simulink library "inp"  (R2021b)
settings: Solver=VariableStepAuto  StartTime=0.0  StopTime=10.0  RelTol=1e-3
undefined symbols (not defined in the file): C_TASK_5MS_S, FALSE, KINP_AcoreReadyToSlp_flg_ovrdflg, KINP_AcoreReadyToSlp_flg_ovrdval, KINP_AllowMovThd_OTA_enum_ovrdflg, KINP_AllowMovThd_OTA_enum_ovrdval, KINP_APSAngleTarget_Deg_ovrdflg, KINP_APSAngleTarget_Deg_ovrdval, KINP_APSDecReq_mps2_ovrdflg, KINP_APSDecReq_mps2_ovrdval, KINP_APSDecReqA_flg_ovrdflg, KINP_APSDecReqA_flg_ovrdval, KINP_APSDFLL_cm_ovrdflg, KINP_APSDFLL_cm_ovrdval, KINP_APSDFLR_cm_ovrdflg, KINP_APSDFLR_cm_ovrdval, KINP_APSDRLL_cm_ovrdflg, KINP_APSDRLL_cm_ovrdval, KINP_APSDRLR_cm_ovrdflg, KINP_APSDRLR_cm_ovrdval, KINP_APSExitCondition_enum_ovrdflg, KINP_APSExitCondition_enum_ovrdval, KINP_APSHWVer_enum_ovrdflg, KINP_APSHWVer_enum_ovrdval, KINP_APSProgressPCT_pct_ovrdflg, KINP_APSProgressPCT_pct_ovrdval, KINP_APSReq_enum_ovrdflg, KINP_APSReq_enum_ovrdval, KINP_APSRQDisplay_enum_ovrdflg, KINP_APSRQDisplay_enum_ovrdval, KINP_APSRqEPASCtrl_flg_ovrdflg, KINP_APSRqEPASCtrl_flg_ovrdval, KINP_APSShiftPosnReq_enum_ovrdval, KINP_APSShiftPosnReq_enum_ovrflg, KINP_APSSpeedCMD_kph_ovrdval, KINP_APSSpeedCMD_kph_ovrflg, KINP_APSStaSystem_enum_ovrdflg, KINP_APSStaSystem_enum_ovrdval, KINP_APSSWVer_enum_ovrdflg, KINP_APSSWVer_enum_ovrdval, KINP_APSVMCReqA_flg_ovrdval, KINP_APSVMCReqA_flg_ovrflg, KINP_APSVRqEPASCtrl_flg_ovrdflg, KINP_APSVRqEPASCtrl_flg_ovrdval, KINP_AuxBattVolmV_mV_ovrdflg, KINP_AuxBattVolmV_mV_ovrdval, KINP_CAASSta_enum_ovrdflg, KINP_CAASSta_enum_ovrdval, KINP_CAASVMCReqA_flg_ovrdval, KINP_CAASVMCReqA_flg_ovrflg, KINP_Chime_enum_ovrdflg, KINP_Chime_enum_ovrdval, KINP_ClearDTCcmd_flg_ovrdflg, KINP_ClearDTCcmd_flg_ovrdval, KINP_EvccAplusPwrUpReq_flg_ovrdflg, KINP_EvccAplusPwrUpReq_flg_ovrdval, KINP_LFID_raw_ovrdval, KINP_LFID_raw_ovrflg, KINP_LRID_raw_ovrdval, KINP_MemOffsetAccX_raw16_ovrdflg ... (+118)
libraries: FVT_lib x595, hcu_lib x1
(part 23 of 27)

== system inp/INP/CAN4/SignalCheck/GW_ZoneDR1 ==
  BHAL_outputs : Inport
  inp_CanValid_bus : Inport  Port=2
  CSWDimSw : FVT_lib/inp/can_signal_template  SystemSampleTime=-1  VariantActivationTime=update diagram  Latency=0  AutoFrameSizeCalculation=off
      link override defval: Value=KINP_CSWDimSw_flg_defval
      link override fftdec: Value=KINP_CSWDimSw_flg_fftdec
      link override fftinc: Value=KINP_CSWDimSw_flg_fftinc
      link override fftlim: Value=KINP_CSWDimSw_flg_fftlim
      link override invalid: Value=KINP_CSWDimSw_flg_invalid
      link override ovrdflg: Value=KINP_CSWDimSw_flg_ovrdflg
      link override ovrdval: Value=KINP_CSWDimSw_flg_ovrdval
      link override setvalid: Value=KINP_CSWDimSw_flg_setvalid
      link override srvcflg: Value=KINP_CSWDimSw_flg_srvcflg
      link override srvcval: Value=KINP_CSWDimSw_flg_srvcval
  CSWFWasSwSta : FVT_lib/inp/can_signal_template  SystemSampleTime=-1  VariantActivationTime=update diagram  Latency=0  AutoFrameSizeCalculation=off
      link override defval: Value=KINP_CSWFWasSwSta_enum_defval
      link override fftdec: Value=KINP_CSWFWasSwSta_enum_fftdec
      link override fftinc: Value=KINP_CSWFWasSwSta_enum_fftinc
      link override fftlim: Value=KINP_CSWFWasSwSta_enum_fftlim
      link override invalid: Value=KINP_CSWFWasSwSta_enum_invalid
      link override ovrdflg: Value=KINP_CSWFWasSwSta_enum_ovrdflg
      link override ovrdval: Value=KINP_CSWFWasSwSta_enum_ovrdval
      link override setvalid: Value=KINP_CSWFWasSwSta_enum_setvalid
      link override srvcflg: Value=KINP_CSWFWasSwSta_enum_srvcflg
      link override srvcval: Value=KINP_CSWFWasSwSta_enum_srvcval
  CSWFWipSwSta : FVT_lib/inp/can_signal_template  SystemSampleTime=-1  VariantActivationTime=update diagram  Latency=0  AutoFrameSizeCalculation=off
      link override defval: Value=KINP_CSWFWipSwSta_enum_defval
      link override fftdec: Value=KINP_CSWFWipSwSta_enum_fftdec
      link override fftinc: Value=KINP_CSWFWipSwSta_enum_fftinc
      link override fftlim: Value=KINP_CSWFWipSwSta_enum_fftlim
      link override invalid: Value=KINP_CSWFWipSwSta_enum_invalid
      link override ovrdflg: Value=KINP_CSWFWipSwSta_enum_ovrdflg
      link override ovrdval: Value=KINP_CSWFWipSwSta_enum_ovrdval
      link override setvalid: Value=KINP_CSWFWipSwSta_enum_setvalid
      link override srvcflg: Value=KINP_CSWFWipSwSta_enum_srvcflg
      link override srvcval: Value=KINP_CSWFWipSwSta_enum_srvcval
  CSWPassSWSta : FVT_lib/inp/can_signal_template  SystemSampleTime=-1  VariantActivationTime=update diagram  Latency=0  AutoFrameSizeCalculation=off
      link override defval: Value=KINP_CSWPassSWSta_flg_defval
      link override fftdec: Value=KINP_CSWPassSWSta_flg_fftdec
      link override fftinc: Value=KINP_CSWPassSWSta_flg_fftinc
      link override fftlim: Value=KINP_CSWPassSWSta_flg_fftlim
      link override invalid: Value=KINP_CSWPassSWSta_flg_invalid
      link override ovrdflg: Value=KINP_CSWPassSWSta_flg_ovrdflg
      link override ovrdval: Value=KINP_CSWPassSWSta_flg_ovrdval
      link override setvalid: Value=KINP_CSWPassSWSta_flg_setvalid
      link override srvcflg: Value=KINP_CSWPassSWSta_flg_srvcflg
      link override srvcval: Value=KINP_CSWPassSWSta_flg_srvcval
  CSWRWasSWSta : FVT_lib/inp/can_signal_template  SystemSampleTime=-1  VariantActivationTime=update diagram  Latency=0  AutoFrameSizeCalculation=off
      link override defval: Value=KINP_CSWRWasSWSta_enum_defval
      link override fftdec: Value=KINP_CSWRWasSWSta_enum_fftdec
      link override fftinc: Value=KINP_CSWRWasSWSta_enum_fftinc
      link override fftlim: Value=KINP_CSWRWasSWSta_enum_fftlim
      link override invalid: Value=KINP_CSWRWasSWSta_enum_invalid
      link override ovrdflg: Value=KINP_CSWRWasSWSta_enum_ovrdflg
      link override ovrdval: Value=KINP_CSWRWasSWSta_enum_ovrdval
      link override setvalid: Value=KINP_CSWRWasSWSta_enum_setvalid
      link override srvcflg: Value=KINP_CSWRWasSWSta_enum_srvcflg
      link override srvcval: Value=KINP_CSWRWasSWSta_enum_srvcval
  CSWRWipIntSwSta : FVT_lib/inp/can_signal_template  SystemSampleTime=-1  VariantActivationTime=update diagram  Latency=0  AutoFrameSizeCalculation=off
      link override defval: Value=KINP_CSWRWipIntSwSta_enum_defval
      link override fftdec: Value=KINP_CSWRWipIntSwSta_enum_fftdec
      link override fftinc: Value=KINP_CSWRWipIntSwSta_enum_fftinc
      link override fftlim: Value=KINP_CSWRWipIntSwSta_enum_fftlim
      link override invalid: Value=KINP_CSWRWipIntSwSta_enum_invalid
      link override ovrdflg: Value=KINP_CSWRWipIntSwSta_enum_ovrdflg
      link override ovrdval: Value=KINP_CSWRWipIntSwSta_enum_ovrdval
      link override setvalid: Value=KINP_CSWRWipIntSwSta_enum_setvalid
      link override srvcflg: Value=KINP_CSWRWipIntSwSta_enum_srvcflg
      link override srvcval: Value=KINP_CSWRWipIntSwSta_enum_srvcval
  CSWTurnSwSta : FVT_lib/inp/can_signal_template  SystemSampleTime=-1  VariantActivationTime=update diagram  Latency=0  AutoFrameSizeCalculation=off
      link override defval: Value=KINP_CSWTurnSwSta_enum_defval
      link override fftdec: Value=KINP_CSWTurnSwSta_enum_fftdec
      link override fftinc: Value=KINP_CSWTurnSwSta_enum_fftinc
      link override fftlim: Value=KINP_CSWTurnSwSta_enum_fftlim
      link override invalid: Value=KINP_CSWTurnSwSta_enum_invalid
      link override ovrdflg: Value=KINP_CSWTurnSwSta_enum_ovrdflg
      link override ovrdval: Value=KINP_CSWTurnSwSta_enum_ovrdval
      link override setvalid: Value=KINP_CSWTurnSwSta_enum_setvalid
      link override srvcflg: Value=KINP_CSWTurnSwSta_enum_srvcflg
      link override srvcval: Value=KINP_CSWTurnSwSta_enum_srvcval
  DrLockSta : FVT_lib/inp/can_signal_template  SystemSampleTime=-1  VariantActivationTime=update diagram  Latency=0  AutoFrameSizeCalculation=off
      link override defval: Value=KINP_DrLockSta_flg_defval
      link override fftdec: Value=KINP_DrLockSta_flg_fftdec
      link override fftinc: Value=KINP_DrLockSta_flg_fftinc
      link override fftlim: Value=KINP_DrLockSta_flg_fftlim
      link override invalid: Value=KINP_DrLockSta_flg_invalid
      link override ovrdflg: Value=KINP_DrLockSta_flg_ovrdflg
      link override ovrdval: Value=KINP_DrLockSta_flg_ovrdval
      link override setvalid: Value=KINP_DrLockSta_flg_setvalid
      link override srvcflg: Value=KINP_DrLockSta_flg_srvcflg
      link override srvcval: Value=KINP_DrLockSta_flg_srvcval
  MIRRORFOLDSW : FVT_lib/inp/can_signal_template  SystemSampleTime=-1  VariantActivationTime=update diagram  Latency=0  AutoFrameSizeCalculation=off
      link override defval: Value=KINP_MIRRORFOLDSW_flg_defval
      link override fftdec: Value=KINP_MIRRORFOLDSW_flg_fftdec
      link override fftinc: Value=KINP_MIRRORFOLDSW_flg_fftinc
      link override fftlim: Value=KINP_MIRRORFOLDSW_flg_fftlim
      link override invalid: Value=KINP_MIRRORFOLDSW_flg_invalid
      link override ovrdflg: Value=KINP_MIRRORFOLDSW_flg_ovrdflg
      link override ovrdval: Value=KINP_MIRRORFOLDSW_flg_ovrdval
      link override setvalid: Value=KINP_MIRRORFOLDSW_flg_setvalid
      link override srvcflg: Value=KINP_MIRRORFOLDSW_flg_srvcflg
      link override srvcval: Value=KINP_MIRRORFOLDSW_flg_srvcval
  RLSLampSta : FVT_lib/inp/can_signal_template  SystemSampleTime=-1  VariantActivationTime=update diagram  Latency=0  AutoFrameSizeCalculation=off
      link override defval: Value=KINP_RLSLampSta_flg_defval
      link override fftdec: Value=KINP_RLSLampSta_flg_fftdec
      link override fftinc: Value=KINP_RLSLampSta_flg_fftinc
      link override fftlim: Value=KINP_RLSLampSta_flg_fftlim
      link override invalid: Value=KINP_RLSLampSta_flg_invalid
      link override ovrdflg: Value=KINP_RLSLampSta_flg_ovrdflg
      link override ovrdval: Value=KINP_RLSLampSta_flg_ovrdval
      link override setvalid: Value=KINP_RLSLampSta_flg_setvalid
      link override srvcflg: Value=KINP_RLSLampSta_flg_srvcflg
      link override srvcval: Value=KINP_RLSLampSta_flg_srvcval
  RLSRainSnrWiperCmd : FVT_lib/inp/can_signal_template  SystemSampleTime=-1  VariantActivationTime=update diagram  Latency=0  AutoFrameSizeCalculation=off
      link override defval: Value=KINP_RLSRainSnrWiperCmd_enum_defval
      link override fftdec: Value=KINP_RLSRainSnrWiperCmd_enum_fftdec
      link override fftinc: Value=KINP_RLSRainSnrWiperCmd_enum_fftinc
      link override fftlim: Value=KINP_RLSRainSnrWiperCmd_enum_fftlim
      link override invalid: Value=KINP_RLSRainSnrWiperCmd_enum_invalid
      link override ovrdflg: Value=KINP_RLSRainSnrWiperCmd_enum_ovrdflg
      link override ovrdval: Value=KINP_RLSRainSnrWiperCmd_enum_ovrdval
      link override setvalid: Value=KINP_RLSRainSnrWiperCmd_enum_setvalid
      link override srvcflg: Value=KINP_RLSRainSnrWiperCmd_enum_srvcflg
      link override srvcval: Value=KINP_RLSRainSnrWiperCmd_enum_srvcval
  RLTurnLampC : FVT_lib/inp/can_signal_template  SystemSampleTime=-1  VariantActivationTime=update diagram  Latency=0  AutoFrameSizeCalculation=off
      link override defval: Value=KINP_RLTurnLampC_mA_defval
      link override fftdec: Value=KINP_RLTurnLampC_mA_fftdec
      link override fftinc: Value=KINP_RLTurnLampC_mA_fftinc
      link override fftlim: Value=KINP_RLTurnLampC_mA_fftlim
      link override invalid: Value=KINP_RLTurnLampC_mA_invalid
      link override ovrdflg: Value=KINP_RLTurnLampC_mA_ovrdflg
      link override ovrdval: Value=KINP_RLTurnLampC_mA_ovrdval
      link override setvalid: Value=KINP_RLTurnLampC_mA_setvalid
      link override srvcflg: Value=KINP_RLTurnLampC_mA_srvcflg
      link override srvcval: Value=KINP_RLTurnLampC_mA_srvcval
  RRTurnLampC : FVT_lib/inp/can_signal_template  SystemSampleTime=-1  VariantActivationTime=update diagram  Latency=0  AutoFrameSizeCalculation=off
      link override defval: Value=KINP_RRTurnLampC_mA_defval
      link override fftdec: Value=KINP_RRTurnLampC_mA_fftdec
      link override fftinc: Value=KINP_RRTurnLampC_mA_fftinc
      link override fftlim: Value=KINP_RRTurnLampC_mA_fftlim
      link override invalid: Value=KINP_RRTurnLampC_mA_invalid
      link override ovrdflg: Value=KINP_RRTurnLampC_mA_ovrdflg
      link override ovrdval: Value=KINP_RRTurnLampC_mA_ovrdval
      link override setvalid: Value=KINP_RRTurnLampC_mA_setvalid
      link override srvcflg: Value=KINP_RRTurnLampC_mA_srvcflg
      link override srvcval: Value=KINP_RRTurnLampC_mA_srvcval
  RWiperAS : FVT_lib/inp/can_signal_template  SystemSampleTime=-1  VariantActivationTime=update diagram  Latency=0  AutoFrameSizeCalculation=off
      link override defval: Value=KINP_RWiperAS_flg_defval
      link override fftdec: Value=KINP_RWiperAS_flg_fftdec
      link override fftinc: Value=KINP_RWiperAS_flg_fftinc
      link override fftlim: Value=KINP_RWiperAS_flg_fftlim
      link override invalid: Value=KINP_RWiperAS_flg_invalid
      link override ovrdflg: Value=KINP_RWiperAS_flg_ovrdflg
      link override ovrdval: Value=KINP_RWiperAS_flg_ovrdval
      link override setvalid: Value=KINP_RWiperAS_flg_setvalid
      link override srvcflg: Value=KINP_RWiperAS_flg_srvcflg
      link override srvcval: Value=KINP_RWiperAS_flg_srvcval
  RWiperProtection : FVT_lib/inp/can_signal_template  SystemSampleTime=-1  VariantActivationTime=update diagram  Latency=0  AutoFrameSizeCalculation=off
      link override defval: Value=KINP_RWiperProtection_flg_defval
      link override fftdec: Value=KINP_RWiperProtection_flg_fftdec
      link override fftinc: Value=KINP_RWiperProtection_flg_fftinc
      link override fftlim: Value=KINP_RWiperProtection_flg_fftlim
      link override invalid: Value=KINP_RWiperProtection_flg_invalid
      link override ovrdflg: Value=KINP_RWiperProtection_flg_ovrdflg
      link override ovrdval: Value=KINP_RWiperProtection_flg_ovrdval
      link override setvalid: Value=KINP_RWiperProtection_flg_setvalid
      link override srvcflg: Value=KINP_RWiperProtection_flg_srvcflg
      link override srvcval: Value=KINP_RWiperProtection_flg_srvcval
  Terminator_{1..15} (15 alike) : Terminator
  True_VHAL_CSWDimSw_flg : Constant  Value=TRUE  OutDataTypeStr=boolean
  True_VHAL_CSWFWasSwSta_enum : Constant  Value=TRUE  OutDataTypeStr=boolean
  True_VHAL_CSWFWipSwSta_enum : Constant  Value=TRUE  OutDataTypeStr=boolean
  True_VHAL_CSWPassSWSta_flg : Constant  Value=TRUE  OutDataTypeStr=boolean
  True_VHAL_CSWRWasSWSta_enum : Constant  Value=TRUE  OutDataTypeStr=boolean
  True_VHAL_CSWRWipIntSwSta_enum : Constant  Value=TRUE  OutDataTypeStr=boolean
  True_VHAL_CSWTurnSwSta_enum : Constant  Value=TRUE  OutDataTypeStr=boolean
  True_VHAL_DrLockSta_flg : Constant  Value=TRUE  OutDataTypeStr=boolean
  True_VHAL_MIRRORFOLDSW_flg : Constant  Value=TRUE  OutDataTypeStr=boolean
  True_VHAL_RLSLampSta_flg : Constant  Value=TRUE  OutDataTypeStr=boolean
  True_VHAL_RLSRainSnrWiperCmd_enum : Constant  Value=TRUE  OutDataTypeStr=boolean
  True_VHAL_RLTurnLampC_mA : Constant  Value=TRUE  OutDataTypeStr=boolean
  True_VHAL_RRTurnLampC_mA : Constant  Value=TRUE  OutDataTypeStr=boolean
  True_VHAL_RWiperAS_flg : Constant  Value=TRUE  OutDataTypeStr=boolean
  True_VHAL_RWiperProtection_flg : Constant  Value=TRUE  OutDataTypeStr=boolean
  slr1_{1..15} (15 alike) : BusSelector  OutputSignals=VINP_CANMsgValidGWZoneDR1_flg
  slr_VHAL_CSWDimSw_flg : BusSelector  OutputSignals=VHAL_CSWDimSw_flg
  slr_VHAL_CSWFWasSwSta_enum : BusSelector  OutputSignals=VHAL_CSWFWasSwSta_enum
  slr_VHAL_CSWFWipSwSta_enum : BusSelector  OutputSignals=VHAL_CSWFWipSwSta_enum
  slr_VHAL_CSWPassSWSta_flg : BusSelector  OutputSignals=VHAL_CSWPassSWSta_flg
  slr_VHAL_CSWRWasSWSta_enum : BusSelector  OutputSignals=VHAL_CSWRWasSWSta_enum
  slr_VHAL_CSWRWipIntSwSta_enum : BusSelector  OutputSignals=VHAL_CSWRWipIntSwSta_enum
  slr_VHAL_CSWTurnSwSta_enum : BusSelector  OutputSignals=VHAL_CSWTurnSwSta_enum
  slr_VHAL_DrLockSta_flg : BusSelector  OutputSignals=VHAL_DrLockSta_flg
  slr_VHAL_MIRRORFOLDSW_flg : BusSelector  OutputSignals=VHAL_MIRRORFOLDSW_flg
  slr_VHAL_RLSLampSta_flg : BusSelector  OutputSignals=VHAL_RLSLampSta_flg
  slr_VHAL_RLSRainSnrWiperCmd_enum : BusSelector  OutputSignals=VHAL_RLSRainSnrWiperCmd_enum
  slr_VHAL_RLTurnLampC_mA : BusSelector  OutputSignals=VHAL_RLTurnLampC_mA
  slr_VHAL_RRTurnLampC_mA : BusSelector  OutputSignals=VHAL_RRTurnLampC_mA
  slr_VHAL_RWiperAS_flg : BusSelector  OutputSignals=VHAL_RWiperAS_flg
  slr_VHAL_RWiperProtection_flg : BusSelector  OutputSignals=VHAL_RWiperProtection_flg
  VINP_CSWDimSw_flg : Outport
  VINP_CSWFWasSwSta_enum : Outport  Port=2
  VINP_CSWFWipSwSta_enum : Outport  Port=3
  VINP_CSWPassSWSta_flg : Outport  Port=4
  VINP_CSWRWasSWSta_enum : Outport  Port=5
  VINP_CSWRWipIntSwSta_enum : Outport  Port=6
  VINP_CSWTurnSwSta_enum : Outport  Port=7
  VINP_DrLockSta_flg : Outport  Port=8
  VINP_MIRRORFOLDSW_flg : Outport  Port=9
  VINP_RLSLampSta_flg : Outport  Port=10
  VINP_RLSRainSnrWiperCmd_enum : Outport  Port=11
  VINP_RLTurnLampC_mA : Outport  Port=12
  VINP_RRTurnLampC_mA : Outport  Port=13
  VINP_RWiperAS_flg : Outport  Port=14
  VINP_RWiperProtection_flg : Outport  Port=15
  wires:
  BHAL_outputs/1 -> [BHAL_outputs]
  inp_CanValid_bus/1 -> [inp_CanValid_bus]
  [BHAL_outputs] -> slr_VHAL_CSWDimSw_flg/1
  slr_VHAL_CSWDimSw_flg/1 -> CSWDimSw/1  "<VHAL_CSWDimSw_flg>"
  True_VHAL_CSWDimSw_flg/1 -> CSWDimSw/2
  [inp_CanValid_bus] -> slr1_1/1
  slr1_1/1 -> CSWDimSw/3  "<VINP_CANMsgValidGWZoneDR1_flg>"
  CSWDimSw/1 -> VINP_CSWDimSw_flg/1  "VINP_CSWDimSw_flg"
  CSWDimSw/2 -> Terminator_1/1
  [BHAL_outputs] -> slr_VHAL_CSWFWasSwSta_enum/1
  slr_VHAL_CSWFWasSwSta_enum/1 -> CSWFWasSwSta/1  "<VHAL_CSWFWasSwSta_enum>"
  True_VHAL_CSWFWasSwSta_enum/1 -> CSWFWasSwSta/2
  [inp_CanValid_bus] -> slr1_2/1
  slr1_2/1 -> CSWFWasSwSta/3  "<VINP_CANMsgValidGWZoneDR1_flg>"
  CSWFWasSwSta/1 -> VINP_CSWFWasSwSta_enum/1  "VINP_CSWFWasSwSta_enum"
  CSWFWasSwSta/2 -> Terminator_2/1
  [BHAL_outputs] -> slr_VHAL_CSWFWipSwSta_enum/1
  slr_VHAL_CSWFWipSwSta_enum/1 -> CSWFWipSwSta/1  "<VHAL_CSWFWipSwSta_enum>"
  True_VHAL_CSWFWipSwSta_enum/1 -> CSWFWipSwSta/2
  [inp_CanValid_bus] -> slr1_3/1
  slr1_3/1 -> CSWFWipSwSta/3  "<VINP_CANMsgValidGWZoneDR1_flg>"
  CSWFWipSwSta/1 -> VINP_CSWFWipSwSta_enum/1  "VINP_CSWFWipSwSta_enum"
  CSWFWipSwSta/2 -> Terminator_3/1
  [BHAL_outputs] -> slr_VHAL_CSWPassSWSta_flg/1
  slr_VHAL_CSWPassSWSta_flg/1 -> CSWPassSWSta/1  "<VHAL_CSWPassSWSta_flg>"
  True_VHAL_CSWPassSWSta_flg/1 -> CSWPassSWSta/2
  [inp_CanValid_bus] -> slr1_4/1
  slr1_4/1 -> CSWPassSWSta/3  "<VINP_CANMsgValidGWZoneDR1_flg>"
  CSWPassSWSta/1 -> VINP_CSWPassSWSta_flg/1  "VINP_CSWPassSWSta_flg"
  CSWPassSWSta/2 -> Terminator_4/1
  [BHAL_outputs] -> slr_VHAL_CSWRWasSWSta_enum/1
  slr_VHAL_CSWRWasSWSta_enum/1 -> CSWRWasSWSta/1  "<VHAL_CSWRWasSWSta_enum>"
  True_VHAL_CSWRWasSWSta_enum/1 -> CSWRWasSWSta/2
  [inp_CanValid_bus] -> slr1_5/1
  slr1_5/1 -> CSWRWasSWSta/3  "<VINP_CANMsgValidGWZoneDR1_flg>"
  CSWRWasSWSta/1 -> VINP_CSWRWasSWSta_enum/1  "VINP_CSWRWasSWSta_enum"
  CSWRWasSWSta/2 -> Terminator_5/1
  [BHAL_outputs] -> slr_VHAL_CSWRWipIntSwSta_enum/1
  slr_VHAL_CSWRWipIntSwSta_enum/1 -> CSWRWipIntSwSta/1  "<VHAL_CSWRWipIntSwSta_enum>"
  True_VHAL_CSWRWipIntSwSta_enum/1 -> CSWRWipIntSwSta/2
  [inp_CanValid_bus] -> slr1_6/1
  slr1_6/1 -> CSWRWipIntSwSta/3  "<VINP_CANMsgValidGWZoneDR1_flg>"
  CSWRWipIntSwSta/1 -> VINP_CSWRWipIntSwSta_enum/1  "VINP_CSWRWipIntSwSta_enum"
  CSWRWipIntSwSta/2 -> Terminator_6/1
  [BHAL_outputs] -> slr_VHAL_CSWTurnSwSta_enum/1
  slr_VHAL_CSWTurnSwSta_enum/1 -> CSWTurnSwSta/1  "<VHAL_CSWTurnSwSta_enum>"
  True_VHAL_CSWTurnSwSta_enum/1 -> CSWTurnSwSta/2
  [inp_CanValid_bus] -> slr1_7/1
  slr1_7/1 -> CSWTurnSwSta/3  "<VINP_CANMsgValidGWZoneDR1_flg>"
  CSWTurnSwSta/1 -> VINP_CSWTurnSwSta_enum/1  "VINP_CSWTurnSwSta_enum"
  CSWTurnSwSta/2 -> Terminator_7/1
  [BHAL_outputs] -> slr_VHAL_DrLockSta_flg/1
  slr_VHAL_DrLockSta_flg/1 -> DrLockSta/1  "<VHAL_DrLockSta_flg>"
  True_VHAL_DrLockSta_flg/1 -> DrLockSta/2
  [inp_CanValid_bus] -> slr1_8/1
  slr1_8/1 -> DrLockSta/3  "<VINP_CANMsgValidGWZoneDR1_flg>"
  DrLockSta/1 -> VINP_DrLockSta_flg/1  "VINP_DrLockSta_flg"
  DrLockSta/2 -> Terminator_8/1
  [BHAL_outputs] -> slr_VHAL_MIRRORFOLDSW_flg/1
  slr_VHAL_MIRRORFOLDSW_flg/1 -> MIRRORFOLDSW/1  "<VHAL_MIRRORFOLDSW_flg>"
  True_VHAL_MIRRORFOLDSW_flg/1 -> MIRRORFOLDSW/2
  [inp_CanValid_bus] -> slr1_9/1
  slr1_9/1 -> MIRRORFOLDSW/3  "<VINP_CANMsgValidGWZoneDR1_flg>"
  MIRRORFOLDSW/1 -> VINP_MIRRORFOLDSW_flg/1  "VINP_MIRRORFOLDSW_flg"
  MIRRORFOLDSW/2 -> Terminator_9/1
  [BHAL_outputs] -> slr_VHAL_RLSLampSta_flg/1
  slr_VHAL_RLSLampSta_flg/1 -> RLSLampSta/1  "<VHAL_RLSLampSta_flg>"
  True_VHAL_RLSLampSta_flg/1 -> RLSLampSta/2
  [inp_CanValid_bus] -> slr1_10/1
  slr1_10/1 -> RLSLampSta/3  "<VINP_CANMsgValidGWZoneDR1_flg>"
  RLSLampSta/1 -> VINP_RLSLampSta_flg/1  "VINP_RLSLampSta_flg"
  RLSLampSta/2 -> Terminator_10/1
  [BHAL_outputs] -> slr_VHAL_RLSRainSnrWiperCmd_enum/1
  slr_VHAL_RLSRainSnrWiperCmd_enum/1 -> RLSRainSnrWiperCmd/1  "<VHAL_RLSRainSnrWiperCmd_enum>"
  True_VHAL_RLSRainSnrWiperCmd_enum/1 -> RLSRainSnrWiperCmd/2
  [inp_CanValid_bus] -> slr1_11/1
  slr1_11/1 -> RLSRainSnrWiperCmd/3  "<VINP_CANMsgValidGWZoneDR1_flg>"
  RLSRainSnrWiperCmd/1 -> VINP_RLSRainSnrWiperCmd_enum/1  "VINP_RLSRainSnrWiperCmd_enum"
  RLSRainSnrWiperCmd/2 -> Terminator_11/1
  [BHAL_outputs] -> slr_VHAL_RLTurnLampC_mA/1
  slr_VHAL_RLTurnLampC_mA/1 -> RLTurnLampC/1  "<VHAL_RLTurnLampC_mA>"
  True_VHAL_RLTurnLampC_mA/1 -> RLTurnLampC/2
  [inp_CanValid_bus] -> slr1_12/1
  slr1_12/1 -> RLTurnLampC/3  "<VINP_CANMsgValidGWZoneDR1_flg>"
  RLTurnLampC/1 -> VINP_RLTurnLampC_mA/1  "VINP_RLTurnLampC_mA"
  RLTurnLampC/2 -> Terminator_12/1
  [BHAL_outputs] -> slr_VHAL_RRTurnLampC_mA/1
  slr_VHAL_RRTurnLampC_mA/1 -> RRTurnLampC/1  "<VHAL_RRTurnLampC_mA>"
  True_VHAL_RRTurnLampC_mA/1 -> RRTurnLampC/2
  [inp_CanValid_bus] -> slr1_13/1
  slr1_13/1 -> RRTurnLampC/3  "<VINP_CANMsgValidGWZoneDR1_flg>"
  RRTurnLampC/1 -> VINP_RRTurnLampC_mA/1  "VINP_RRTurnLampC_mA"
  RRTurnLampC/2 -> Terminator_13/1
  [BHAL_outputs] -> slr_VHAL_RWiperAS_flg/1
  slr_VHAL_RWiperAS_flg/1 -> RWiperAS/1  "<VHAL_RWiperAS_flg>"
  True_VHAL_RWiperAS_flg/1 -> RWiperAS/2
  [inp_CanValid_bus] -> slr1_14/1
  slr1_14/1 -> RWiperAS/3  "<VINP_CANMsgValidGWZoneDR1_flg>"
  RWiperAS/1 -> VINP_RWiperAS_flg/1  "VINP_RWiperAS_flg"
  RWiperAS/2 -> Terminator_14/1
  [BHAL_outputs] -> slr_VHAL_RWiperProtection_flg/1
  slr_VHAL_RWiperProtection_flg/1 -> RWiperProtection/1  "<VHAL_RWiperProtection_flg>"
  True_VHAL_RWiperProtection_flg/1 -> RWiperProtection/2
  [inp_CanValid_bus] -> slr1_15/1
  slr1_15/1 -> RWiperProtection/3  "<VINP_CANMsgValidGWZoneDR1_flg>"
  RWiperProtection/1 -> VINP_RWiperProtection_flg/1  "VINP_RWiperProtection_flg"
  RWiperProtection/2 -> Terminator_15/1

== system inp/INP/CAN4/SignalCheck/GW_ZoneDR2 ==
  BHAL_outputs : Inport
  inp_CanValid_bus : Inport  Port=2
  SWCCANCELSta : FVT_lib/inp/can_signal_template  SystemSampleTime=-1  VariantActivationTime=update diagram  Latency=0  AutoFrameSizeCalculation=off
      link override defval: Value=KINP_SWCCANCELSta_flg_defval
      link override fftdec: Value=KINP_SWCCANCELSta_flg_fftdec
      link override fftinc: Value=KINP_SWCCANCELSta_flg_fftinc
      link override fftlim: Value=KINP_SWCCANCELSta_flg_fftlim
      link override invalid: Value=KINP_SWCCANCELSta_flg_invalid
      link override ovrdflg: Value=KINP_SWCCANCELSta_flg_ovrdflg
      link override ovrdval: Value=KINP_SWCCANCELSta_flg_ovrdval
      link override setvalid: Value=KINP_SWCCANCELSta_flg_setvalid
      link override srvcflg: Value=KINP_SWCCANCELSta_flg_srvcflg
      link override srvcval: Value=KINP_SWCCANCELSta_flg_srvcval
  SWCResUpSta : FVT_lib/inp/can_signal_template  SystemSampleTime=-1  VariantActivationTime=update diagram  Latency=0  AutoFrameSizeCalculation=off
      link override defval: Value=KINP_SWCResUpSta_flg_defval
      link override fftdec: Value=KINP_SWCResUpSta_flg_fftdec
      link override fftinc: Value=KINP_SWCResUpSta_flg_fftinc
      link override fftlim: Value=KINP_SWCResUpSta_flg_fftlim
      link override invalid: Value=KINP_SWCResUpSta_flg_invalid
      link override ovrdflg: Value=KINP_SWCResUpSta_flg_ovrdflg
      link override ovrdval: Value=KINP_SWCResUpSta_flg_ovrdval
      link override setvalid: Value=KINP_SWCResUpSta_flg_setvalid
      link override srvcflg: Value=KINP_SWCResUpSta_flg_srvcflg
      link override srvcval: Value=KINP_SWCResUpSta_flg_srvcval
  SWCSetdownSta : FVT_lib/inp/can_signal_template  SystemSampleTime=-1  VariantActivationTime=update diagram  Latency=0  AutoFrameSizeCalculation=off
      link override defval: Value=KINP_SWCSetdownSta_flg_defval
      link override fftdec: Value=KINP_SWCSetdownSta_flg_fftdec
      link override fftinc: Value=KINP_SWCSetdownSta_flg_fftinc
      link override fftlim: Value=KINP_SWCSetdownSta_flg_fftlim
      link override invalid: Value=KINP_SWCSetdownSta_flg_invalid
      link override ovrdflg: Value=KINP_SWCSetdownSta_flg_ovrdflg
      link override ovrdval: Value=KINP_SWCSetdownSta_flg_ovrdval
      link override setvalid: Value=KINP_SWCSetdownSta_flg_setvalid
      link override srvcflg: Value=KINP_SWCSetdownSta_flg_srvcflg
      link override srvcval: Value=KINP_SWCSetdownSta_flg_srvcval
  SWCmodeSta : FVT_lib/inp/can_signal_template  SystemSampleTime=-1  VariantActivationTime=update diagram  Latency=0  AutoFrameSizeCalculation=off
      link override defval: Value=KINP_SWCmodeSta_flg_defval
      link override fftdec: Value=KINP_SWCmodeSta_flg_fftdec
      link override fftinc: Value=KINP_SWCmodeSta_flg_fftinc
      link override fftlim: Value=KINP_SWCmodeSta_flg_fftlim
      link override invalid: Value=KINP_SWCmodeSta_flg_invalid
      link override ovrdflg: Value=KINP_SWCmodeSta_flg_ovrdflg
      link override ovrdval: Value=KINP_SWCmodeSta_flg_ovrdval
      link override setvalid: Value=KINP_SWCmodeSta_flg_setvalid
      link override srvcflg: Value=KINP_SWCmodeSta_flg_srvcflg
      link override srvcval: Value=KINP_SWCmodeSta_flg_srvcval
  Terminator_{1..4} (4 alike) : Terminator
  True_VHAL_SWCCANCELSta_flg : Constant  Value=TRUE  OutDataTypeStr=boolean
  True_VHAL_SWCResUpSta_flg : Constant  Value=TRUE  OutDataTypeStr=boolean
  True_VHAL_SWCSetdownSta_flg : Constant  Value=TRUE  OutDataTypeStr=boolean
  True_VHAL_SWCmodeSta_flg : Constant  Value=TRUE  OutDataTypeStr=boolean
  slr1_{1..4} (4 alike) : BusSelector  OutputSignals=VINP_CANMsgValidGWZoneDR2_flg
  slr_VHAL_SWCCANCELSta_flg : BusSelector  OutputSignals=VHAL_SWCCANCELSta_flg
  slr_VHAL_SWCResUpSta_flg : BusSelector  OutputSignals=VHAL_SWCResUpSta_flg
  slr_VHAL_SWCSetdownSta_flg : BusSelector  OutputSignals=VHAL_SWCSetdownSta_flg
  slr_VHAL_SWCmodeSta_flg : BusSelector  OutputSignals=VHAL_SWCmodeSta_flg
  VINP_SWCCANCELSta_flg : Outport
  VINP_SWCResUpSta_flg : Outport  Port=2
  VINP_SWCSetdownSta_flg : Outport  Port=3
  VINP_SWCmodeSta_flg : Outport  Port=4
  wires:
  BHAL_outputs/1 -> [BHAL_outputs]
  inp_CanValid_bus/1 -> [inp_CanValid_bus]
  [BHAL_outputs] -> slr_VHAL_SWCCANCELSta_flg/1
  slr_VHAL_SWCCANCELSta_flg/1 -> SWCCANCELSta/1  "<VHAL_SWCCANCELSta_flg>"
  True_VHAL_SWCCANCELSta_flg/1 -> SWCCANCELSta/2
  [inp_CanValid_bus] -> slr1_1/1
  slr1_1/1 -> SWCCANCELSta/3  "<VINP_CANMsgValidGWZoneDR2_flg>"
  SWCCANCELSta/1 -> VINP_SWCCANCELSta_flg/1  "VINP_SWCCANCELSta_flg"
  SWCCANCELSta/2 -> Terminator_1/1
  [BHAL_outputs] -> slr_VHAL_SWCResUpSta_flg/1
  slr_VHAL_SWCResUpSta_flg/1 -> SWCResUpSta/1  "<VHAL_SWCResUpSta_flg>"
  True_VHAL_SWCResUpSta_flg/1 -> SWCResUpSta/2
  [inp_CanValid_bus] -> slr1_2/1
  slr1_2/1 -> SWCResUpSta/3  "<VINP_CANMsgValidGWZoneDR2_flg>"
  SWCResUpSta/1 -> VINP_SWCResUpSta_flg/1  "VINP_SWCResUpSta_flg"
  SWCResUpSta/2 -> Terminator_2/1
  [BHAL_outputs] -> slr_VHAL_SWCSetdownSta_flg/1
  slr_VHAL_SWCSetdownSta_flg/1 -> SWCSetdownSta/1  "<VHAL_SWCSetdownSta_flg>"
  True_VHAL_SWCSetdownSta_flg/1 -> SWCSetdownSta/2
  [inp_CanValid_bus] -> slr1_3/1
  slr1_3/1 -> SWCSetdownSta/3  "<VINP_CANMsgValidGWZoneDR2_flg>"
  SWCSetdownSta/1 -> VINP_SWCSetdownSta_flg/1  "VINP_SWCSetdownSta_flg"
  SWCSetdownSta/2 -> Terminator_3/1
  [BHAL_outputs] -> slr_VHAL_SWCmodeSta_flg/1
  slr_VHAL_SWCmodeSta_flg/1 -> SWCmodeSta/1  "<VHAL_SWCmodeSta_flg>"
  True_VHAL_SWCmodeSta_flg/1 -> SWCmodeSta/2
  [inp_CanValid_bus] -> slr1_4/1
  slr1_4/1 -> SWCmodeSta/3  "<VINP_CANMsgValidGWZoneDR2_flg>"
  SWCmodeSta/1 -> VINP_SWCmodeSta_flg/1  "VINP_SWCmodeSta_flg"
  SWCmodeSta/2 -> Terminator_4/1

== system inp/INP/CAN4/SignalCheck/GW_ZoneDR3 ==
  BHAL_outputs : Inport
  inp_CanValid_bus : Inport  Port=2
  LDrvValWdwOpened : FVT_lib/inp/can_signal_template  SystemSampleTime=-1  VariantActivationTime=update diagram  Latency=0  AutoFrameSizeCalculation=off
      link override defval: Value=KINP_LDrvValWdwOpened_pct_defval
      link override fftdec: Value=KINP_LDrvValWdwOpened_pct_fftdec
      link override fftinc: Value=KINP_LDrvValWdwOpened_pct_fftinc
      link override fftlim: Value=KINP_LDrvValWdwOpened_pct_fftlim
      link override invalid: Value=KINP_LDrvValWdwOpened_pct_invalid
      link override ovrdflg: Value=KINP_LDrvValWdwOpened_pct_ovrdflg
      link override ovrdval: Value=KINP_LDrvValWdwOpened_pct_ovrdval
      link override setvalid: Value=KINP_LDrvValWdwOpened_pct_setvalid
      link override srvcflg: Value=KINP_LDrvValWdwOpened_pct_srvcflg
      link override srvcval: Value=KINP_LDrvValWdwOpened_pct_srvcval
  LPasValWdwOpened : FVT_lib/inp/can_signal_template  SystemSampleTime=-1  VariantActivationTime=update diagram  Latency=0  AutoFrameSizeCalculation=off
      link override defval: Value=KINP_LPasValWdwOpened_pct_defval
      link override fftdec: Value=KINP_LPasValWdwOpened_pct_fftdec
      link override fftinc: Value=KINP_LPasValWdwOpened_pct_fftinc
      link override fftlim: Value=KINP_LPasValWdwOpened_pct_fftlim
      link override invalid: Value=KINP_LPasValWdwOpened_pct_invalid
      link override ovrdflg: Value=KINP_LPasValWdwOpened_pct_ovrdflg
      link override ovrdval: Value=KINP_LPasValWdwOpened_pct_ovrdval
      link override setvalid: Value=KINP_LPasValWdwOpened_pct_setvalid
      link override srvcflg: Value=KINP_LPasValWdwOpened_pct_srvcflg
      link override srvcval: Value=KINP_LPasValWdwOpened_pct_srvcval
  Terminator_1 : Terminator
  Terminator_2 : Terminator
  True_VHAL_LDrvValWdwOpened_pct : Constant  Value=TRUE  OutDataTypeStr=boolean
  True_VHAL_LPasValWdwOpened_pct : Constant  Value=TRUE  OutDataTypeStr=boolean
  slr1_1 : BusSelector  OutputSignals=VINP_CANMsgValidGWZoneDR3_flg
  slr1_2 : BusSelector  OutputSignals=VINP_CANMsgValidGWZoneDR3_flg
  slr_VHAL_LDrvValWdwOpened_pct : BusSelector  OutputSignals=VHAL_LDrvValWdwOpened_pct
  slr_VHAL_LPasValWdwOpened_pct : BusSelector  OutputSignals=VHAL_LPasValWdwOpened_pct
  VINP_LDrvValWdwOpened_pct : Outport
  VINP_LPasValWdwOpened_pct : Outport  Port=2
  wires:
  BHAL_outputs/1 -> [BHAL_outputs]
  inp_CanValid_bus/1 -> [inp_CanValid_bus]
  [BHAL_outputs] -> slr_VHAL_LDrvValWdwOpened_pct/1
  slr_VHAL_LDrvValWdwOpened_pct/1 -> LDrvValWdwOpened/1  "<VHAL_LDrvValWdwOpened_pct>"
  True_VHAL_LDrvValWdwOpened_pct/1 -> LDrvValWdwOpened/2
  [inp_CanValid_bus] -> slr1_1/1
  slr1_1/1 -> LDrvValWdwOpened/3  "<VINP_CANMsgValidGWZoneDR3_flg>"
  LDrvValWdwOpened/1 -> VINP_LDrvValWdwOpened_pct/1  "VINP_LDrvValWdwOpened_pct"
  LDrvValWdwOpened/2 -> Terminator_1/1
  [BHAL_outputs] -> slr_VHAL_LPasValWdwOpened_pct/1
  slr_VHAL_LPasValWdwOpened_pct/1 -> LPasValWdwOpened/1  "<VHAL_LPasValWdwOpened_pct>"
  True_VHAL_LPasValWdwOpened_pct/1 -> LPasValWdwOpened/2
  [inp_CanValid_bus] -> slr1_2/1
  slr1_2/1 -> LPasValWdwOpened/3  "<VINP_CANMsgValidGWZoneDR3_flg>"
  LPasValWdwOpened/1 -> VINP_LPasValWdwOpened_pct/1  "VINP_LPasValWdwOpened_pct"
  LPasValWdwOpened/2 -> Terminator_2/1

== system inp/INP/CAN4/SignalCheck/GW_ZoneDR4 ==
  BHAL_outputs : Inport
  inp_CanValid_bus : Inport  Port=2
  LRLDValWdwOpened : FVT_lib/inp/can_signal_template  SystemSampleTime=-1  VariantActivationTime=update diagram  Latency=0  AutoFrameSizeCalculation=off
      link override defval: Value=KINP_LRLDValWdwOpened_pct_defval
      link override fftdec: Value=KINP_LRLDValWdwOpened_pct_fftdec
      link override fftinc: Value=KINP_LRLDValWdwOpened_pct_fftinc
      link override fftlim: Value=KINP_LRLDValWdwOpened_pct_fftlim
      link override invalid: Value=KINP_LRLDValWdwOpened_pct_invalid
      link override ovrdflg: Value=KINP_LRLDValWdwOpened_pct_ovrdflg
      link override ovrdval: Value=KINP_LRLDValWdwOpened_pct_ovrdval
      link override setvalid: Value=KINP_LRLDValWdwOpened_pct_setvalid
      link override srvcflg: Value=KINP_LRLDValWdwOpened_pct_srvcflg
      link override srvcval: Value=KINP_LRLDValWdwOpened_pct_srvcval
  LRRDValWdwOpened : FVT_lib/inp/can_signal_template  SystemSampleTime=-1  VariantActivationTime=update diagram  Latency=0  AutoFrameSizeCalculation=off
      link override defval: Value=KINP_LRRDValWdwOpened_pct_defval
      link override fftdec: Value=KINP_LRRDValWdwOpened_pct_fftdec
      link override fftinc: Value=KINP_LRRDValWdwOpened_pct_fftinc
      link override fftlim: Value=KINP_LRRDValWdwOpened_pct_fftlim
      link override invalid: Value=KINP_LRRDValWdwOpened_pct_invalid
      link override ovrdflg: Value=KINP_LRRDValWdwOpened_pct_ovrdflg
      link override ovrdval: Value=KINP_LRRDValWdwOpened_pct_ovrdval
      link override setvalid: Value=KINP_LRRDValWdwOpened_pct_setvalid
      link override srvcflg: Value=KINP_LRRDValWdwOpened_pct_srvcflg
      link override srvcval: Value=KINP_LRRDValWdwOpened_pct_srvcval
  PTGInnerSW2 : FVT_lib/inp/can_signal_template  SystemSampleTime=-1  VariantActivationTime=update diagram  Latency=0  AutoFrameSizeCalculation=off
      link override defval: Value=KINP_PTGInnerSW2_enum_defval
      link override fftdec: Value=KINP_PTGInnerSW2_enum_fftdec
      link override fftinc: Value=KINP_PTGInnerSW2_enum_fftinc
      link override fftlim: Value=KINP_PTGInnerSW2_enum_fftlim
      link override invalid: Value=KINP_PTGInnerSW2_enum_invalid
      link override ovrdflg: Value=KINP_PTGInnerSW2_enum_ovrdflg
      link override ovrdval: Value=KINP_PTGInnerSW2_enum_ovrdval
      link override setvalid: Value=KINP_PTGInnerSW2_enum_setvalid
      link override srvcflg: Value=KINP_PTGInnerSW2_enum_srvcflg
      link override srvcval: Value=KINP_PTGInnerSW2_enum_srvcval
  Terminator_1 : Terminator
  Terminator_2 : Terminator
  Terminator_3 : Terminator
  True_VHAL_LRLDValWdwOpened_pct : Constant  Value=TRUE  OutDataTypeStr=boolean
  True_VHAL_LRRDValWdwOpened_pct : Constant  Value=TRUE  OutDataTypeStr=boolean
  True_VHAL_PTGInnerSW2_enum : Constant  Value=TRUE  OutDataTypeStr=boolean
  slr1_1 : BusSelector  OutputSignals=VINP_CANMsgValidGWZoneDR4_flg
  slr1_2 : BusSelector  OutputSignals=VINP_CANMsgValidGWZoneDR4_flg
  slr1_3 : BusSelector  OutputSignals=VINP_CANMsgValidGWZoneDR4_flg
  slr_VHAL_LRLDValWdwOpened_pct : BusSelector  OutputSignals=VHAL_LRLDValWdwOpened_pct
  slr_VHAL_LRRDValWdwOpened_pct : BusSelector  OutputSignals=VHAL_LRRDValWdwOpened_pct
  slr_VHAL_PTGInnerSW2_enum : BusSelector  OutputSignals=VHAL_PTGInnerSW2_enum
  VINP_LRLDValWdwOpened_pct : Outport
  VINP_LRRDValWdwOpened_pct : Outport  Port=2
  VINP_PTGInnerSW2_enum : Outport  Port=3
  wires:
  BHAL_outputs/1 -> [BHAL_outputs]
  inp_CanValid_bus/1 -> [inp_CanValid_bus]
  [BHAL_outputs] -> slr_VHAL_LRLDValWdwOpened_pct/1
  slr_VHAL_LRLDValWdwOpened_pct/1 -> LRLDValWdwOpened/1  "<VHAL_LRLDValWdwOpened_pct>"
  True_VHAL_LRLDValWdwOpened_pct/1 -> LRLDValWdwOpened/2
  [inp_CanValid_bus] -> slr1_1/1
  slr1_1/1 -> LRLDValWdwOpened/3  "<VINP_CANMsgValidGWZoneDR4_flg>"
  LRLDValWdwOpened/1 -> VINP_LRLDValWdwOpened_pct/1  "VINP_LRLDValWdwOpened_pct"
  LRLDValWdwOpened/2 -> Terminator_1/1
  [BHAL_outputs] -> slr_VHAL_LRRDValWdwOpened_pct/1
  slr_VHAL_LRRDValWdwOpened_pct/1 -> LRRDValWdwOpened/1  "<VHAL_LRRDValWdwOpened_pct>"
  True_VHAL_LRRDValWdwOpened_pct/1 -> LRRDValWdwOpened/2
  [inp_CanValid_bus] -> slr1_2/1
  slr1_2/1 -> LRRDValWdwOpened/3  "<VINP_CANMsgValidGWZoneDR4_flg>"
  LRRDValWdwOpened/1 -> VINP_LRRDValWdwOpened_pct/1  "VINP_LRRDValWdwOpened_pct"
  LRRDValWdwOpened/2 -> Terminator_2/1
  [BHAL_outputs] -> slr_VHAL_PTGInnerSW2_enum/1
  slr_VHAL_PTGInnerSW2_enum/1 -> PTGInnerSW2/1  "<VHAL_PTGInnerSW2_enum>"
  True_VHAL_PTGInnerSW2_enum/1 -> PTGInnerSW2/2
  [inp_CanValid_bus] -> slr1_3/1
  slr1_3/1 -> PTGInnerSW2/3  "<VINP_CANMsgValidGWZoneDR4_flg>"
  PTGInnerSW2/1 -> VINP_PTGInnerSW2_enum/1  "VINP_PTGInnerSW2_enum"
  PTGInnerSW2/2 -> Terminator_3/1

== system inp/INP/CAN4/SignalCheck/GW_ZoneDR6 ==
  BHAL_outputs : Inport
  inp_CanValid_bus : Inport  Port=2
  FrntPTCRearLeActHeatPwr : FVT_lib/inp/can_signal_template  SystemSampleTime=-1  VariantActivationTime=update diagram  Latency=0  AutoFrameSizeCalculation=off
      link override defval: Value=KINP_FrntPTCRearLeActHeatPwr_W_defval
      link override fftdec: Value=KINP_FrntPTCRearLeActHeatPwr_W_fftdec
      link override fftinc: Value=KINP_FrntPTCRearLeActHeatPwr_W_fftinc
      link override fftlim: Value=KINP_FrntPTCRearLeActHeatPwr_W_fftlim
      link override invalid: Value=KINP_FrntPTCRearLeActHeatPwr_W_invalid
      link override ovrdflg: Value=KINP_FrntPTCRearLeActHeatPwr_W_ovrdflg
      link override ovrdval: Value=KINP_FrntPTCRearLeActHeatPwr_W_ovrdval
      link override setvalid: Value=KINP_FrntPTCRearLeActHeatPwr_W_setvalid
      link override srvcflg: Value=KINP_FrntPTCRearLeActHeatPwr_W_srvcflg
      link override srvcval: Value=KINP_FrntPTCRearLeActHeatPwr_W_srvcval
  FrntPTCRearRiActHeatPwr : FVT_lib/inp/can_signal_template  SystemSampleTime=-1  VariantActivationTime=update diagram  Latency=0  AutoFrameSizeCalculation=off
      link override defval: Value=KINP_FrntPTCRearRiActHeatPwr_W_defval
      link override fftdec: Value=KINP_FrntPTCRearRiActHeatPwr_W_fftdec
      link override fftinc: Value=KINP_FrntPTCRearRiActHeatPwr_W_fftinc
      link override fftlim: Value=KINP_FrntPTCRearRiActHeatPwr_W_fftlim
      link override invalid: Value=KINP_FrntPTCRearRiActHeatPwr_W_invalid
      link override ovrdflg: Value=KINP_FrntPTCRearRiActHeatPwr_W_ovrdflg
      link override ovrdval: Value=KINP_FrntPTCRearRiActHeatPwr_W_ovrdval
      link override setvalid: Value=KINP_FrntPTCRearRiActHeatPwr_W_setvalid
      link override srvcflg: Value=KINP_FrntPTCRearRiActHeatPwr_W_srvcflg
      link override srvcval: Value=KINP_FrntPTCRearRiActHeatPwr_W_srvcval
  FrntPTCRiActHeatPwr : FVT_lib/inp/can_signal_template  SystemSampleTime=-1  VariantActivationTime=update diagram  Latency=0  AutoFrameSizeCalculation=off
      link override defval: Value=KINP_FrntPTCRiActHeatPwr_W_defval
      link override fftdec: Value=KINP_FrntPTCRiActHeatPwr_W_fftdec
      link override fftinc: Value=KINP_FrntPTCRiActHeatPwr_W_fftinc
      link override fftlim: Value=KINP_FrntPTCRiActHeatPwr_W_fftlim
      link override invalid: Value=KINP_FrntPTCRiActHeatPwr_W_invalid
      link override ovrdflg: Value=KINP_FrntPTCRiActHeatPwr_W_ovrdflg
      link override ovrdval: Value=KINP_FrntPTCRiActHeatPwr_W_ovrdval
      link override setvalid: Value=KINP_FrntPTCRiActHeatPwr_W_setvalid
      link override srvcflg: Value=KINP_FrntPTCRiActHeatPwr_W_srvcflg
      link override srvcval: Value=KINP_FrntPTCRiActHeatPwr_W_srvcval
  Terminator_1 : Terminator
  Terminator_2 : Terminator
  Terminator_3 : Terminator
  True_VHAL_FrntPTCRearLeActHeatPwr_W : Constant  Value=TRUE  OutDataTypeStr=boolean
  True_VHAL_FrntPTCRearRiActHeatPwr_W : Constant  Value=TRUE  OutDataTypeStr=boolean
  True_VHAL_FrntPTCRiActHeatPwr_W : Constant  Value=TRUE  OutDataTypeStr=boolean
  slr1_1 : BusSelector  OutputSignals=VINP_CANMsgValidGWZoneDR6_flg
  slr1_2 : BusSelector  OutputSignals=VINP_CANMsgValidGWZoneDR6_flg
  slr1_3 : BusSelector  OutputSignals=VINP_CANMsgValidGWZoneDR6_flg
  slr_VHAL_FrntPTCRearLeActHeatPwr_W : BusSelector  OutputSignals=VHAL_FrntPTCRearLeActHeatPwr_W
  slr_VHAL_FrntPTCRearRiActHeatPwr_W : BusSelector  OutputSignals=VHAL_FrntPTCRearRiActHeatPwr_W
  slr_VHAL_FrntPTCRiActHeatPwr_W : BusSelector  OutputSignals=VHAL_FrntPTCRiActHeatPwr_W
  VINP_FrntPTCRearLeActHeatPwr_W : Outport
  VINP_FrntPTCRearRiActHeatPwr_W : Outport  Port=2
  VINP_FrntPTCRiActHeatPwr_W : Outport  Port=3
  wires:
  BHAL_outputs/1 -> [BHAL_outputs]
  inp_CanValid_bus/1 -> [inp_CanValid_bus]
  [BHAL_outputs] -> slr_VHAL_FrntPTCRearLeActHeatPwr_W/1
  slr_VHAL_FrntPTCRearLeActHeatPwr_W/1 -> FrntPTCRearLeActHeatPwr/1  "<VHAL_FrntPTCRearLeActHeatPwr_W>"
  True_VHAL_FrntPTCRearLeActHeatPwr_W/1 -> FrntPTCRearLeActHeatPwr/2
  [inp_CanValid_bus] -> slr1_1/1
  slr1_1/1 -> FrntPTCRearLeActHeatPwr/3  "<VINP_CANMsgValidGWZoneDR6_flg>"
  FrntPTCRearLeActHeatPwr/1 -> VINP_FrntPTCRearLeActHeatPwr_W/1  "VINP_FrntPTCRearLeActHeatPwr_W"
  FrntPTCRearLeActHeatPwr/2 -> Terminator_1/1
  [BHAL_outputs] -> slr_VHAL_FrntPTCRearRiActHeatPwr_W/1
  slr_VHAL_FrntPTCRearRiActHeatPwr_W/1 -> FrntPTCRearRiActHeatPwr/1  "<VHAL_FrntPTCRearRiActHeatPwr_W>"
  True_VHAL_FrntPTCRearRiActHeatPwr_W/1 -> FrntPTCRearRiActHeatPwr/2
  [inp_CanValid_bus] -> slr1_2/1
  slr1_2/1 -> FrntPTCRearRiActHeatPwr/3  "<VINP_CANMsgValidGWZoneDR6_flg>"
  FrntPTCRearRiActHeatPwr/1 -> VINP_FrntPTCRearRiActHeatPwr_W/1  "VINP_FrntPTCRearRiActHeatPwr_W"
  FrntPTCRearRiActHeatPwr/2 -> Terminator_2/1
  [BHAL_outputs] -> slr_VHAL_FrntPTCRiActHeatPwr_W/1
  slr_VHAL_FrntPTCRiActHeatPwr_W/1 -> FrntPTCRiActHeatPwr/1  "<VHAL_FrntPTCRiActHeatPwr_W>"
  True_VHAL_FrntPTCRiActHeatPwr_W/1 -> FrntPTCRiActHeatPwr/2
  [inp_CanValid_bus] -> slr1_3/1
  slr1_3/1 -> FrntPTCRiActHeatPwr/3  "<VINP_CANMsgValidGWZoneDR6_flg>"
  FrntPTCRiActHeatPwr/1 -> VINP_FrntPTCRiActHeatPwr_W/1  "VINP_FrntPTCRiActHeatPwr_W"
  FrntPTCRiActHeatPwr/2 -> Terminator_3/1

== system inp/INP/CAN4/SignalCheck/GW_ZoneFR1 ==
  BHAL_outputs : Inport
  inp_CanValid_bus : Inport  Port=2
  FLTurnLampC : FVT_lib/inp/can_signal_template  SystemSampleTime=-1  VariantActivationTime=update diagram  Latency=0  AutoFrameSizeCalculation=off
      link override defval: Value=KINP_FLTurnLampC_mA_defval
      link override fftdec: Value=KINP_FLTurnLampC_mA_fftdec
      link override fftinc: Value=KINP_FLTurnLampC_mA_fftinc
      link override fftlim: Value=KINP_FLTurnLampC_mA_fftlim
      link override invalid: Value=KINP_FLTurnLampC_mA_invalid
      link override ovrdflg: Value=KINP_FLTurnLampC_mA_ovrdflg
      link override ovrdval: Value=KINP_FLTurnLampC_mA_ovrdval
      link override setvalid: Value=KINP_FLTurnLampC_mA_setvalid
      link override srvcflg: Value=KINP_FLTurnLampC_mA_srvcflg
      link override srvcval: Value=KINP_FLTurnLampC_mA_srvcval
  FRTurnLampC : FVT_lib/inp/can_signal_template  SystemSampleTime=-1  VariantActivationTime=update diagram  Latency=0  AutoFrameSizeCalculation=off
      link override defval: Value=KINP_FRTurnLampC_mA_defval
      link override fftdec: Value=KINP_FRTurnLampC_mA_fftdec
      link override fftinc: Value=KINP_FRTurnLampC_mA_fftinc
      link override fftlim: Value=KINP_FRTurnLampC_mA_fftlim
      link override invalid: Value=KINP_FRTurnLampC_mA_invalid
      link override ovrdflg: Value=KINP_FRTurnLampC_mA_ovrdflg
      link override ovrdval: Value=KINP_FRTurnLampC_mA_ovrdval
      link override setvalid: Value=KINP_FRTurnLampC_mA_setvalid
      link override srvcflg: Value=KINP_FRTurnLampC_mA_srvcflg
      link override srvcval: Value=KINP_FRTurnLampC_mA_srvcval
  FWiperAS : FVT_lib/inp/can_signal_template  SystemSampleTime=-1  VariantActivationTime=update diagram  Latency=0  AutoFrameSizeCalculation=off
      link override defval: Value=KINP_FWiperAS_flg_defval
      link override fftdec: Value=KINP_FWiperAS_flg_fftdec
      link override fftinc: Value=KINP_FWiperAS_flg_fftinc
      link override fftlim: Value=KINP_FWiperAS_flg_fftlim
      link override invalid: Value=KINP_FWiperAS_flg_invalid
      link override ovrdflg: Value=KINP_FWiperAS_flg_ovrdflg
      link override ovrdval: Value=KINP_FWiperAS_flg_ovrdval
      link override setvalid: Value=KINP_FWiperAS_flg_setvalid
      link override srvcflg: Value=KINP_FWiperAS_flg_srvcflg
      link override srvcval: Value=KINP_FWiperAS_flg_srvcval
  FWiperProtection : FVT_lib/inp/can_signal_template  SystemSampleTime=-1  VariantActivationTime=update diagram  Latency=0  AutoFrameSizeCalculation=off
      link override defval: Value=KINP_FWiperProtection_flg_defval
      link override fftdec: Value=KINP_FWiperProtection_flg_fftdec
      link override fftinc: Value=KINP_FWiperProtection_flg_fftinc
      link override fftlim: Value=KINP_FWiperProtection_flg_fftlim
      link override invalid: Value=KINP_FWiperProtection_flg_invalid
      link override ovrdflg: Value=KINP_FWiperProtection_flg_ovrdflg
      link override ovrdval: Value=KINP_FWiperProtection_flg_ovrdval
      link override setvalid: Value=KINP_FWiperProtection_flg_setvalid
      link override srvcflg: Value=KINP_FWiperProtection_flg_srvcflg
      link override srvcval: Value=KINP_FWiperProtection_flg_srvcval
  Terminator_{1..4} (4 alike) : Terminator
  True_VHAL_FLTurnLampC_mA : Constant  Value=TRUE  OutDataTypeStr=boolean
  True_VHAL_FRTurnLampC_mA : Constant  Value=TRUE  OutDataTypeStr=boolean
  True_VHAL_FWiperAS_flg : Constant  Value=TRUE  OutDataTypeStr=boolean
  True_VHAL_FWiperProtection_flg : Constant  Value=TRUE  OutDataTypeStr=boolean
  slr1_{1..4} (4 alike) : BusSelector  OutputSignals=VINP_CANMsgValidGWZoneFR1_flg
  slr_VHAL_FLTurnLampC_mA : BusSelector  OutputSignals=VHAL_FLTurnLampC_mA
  slr_VHAL_FRTurnLampC_mA : BusSelector  OutputSignals=VHAL_FRTurnLampC_mA
  slr_VHAL_FWiperAS_flg : BusSelector  OutputSignals=VHAL_FWiperAS_flg
  slr_VHAL_FWiperProtection_flg : BusSelector  OutputSignals=VHAL_FWiperProtection_flg
  VINP_FLTurnLampC_mA : Outport
  VINP_FRTurnLampC_mA : Outport  Port=2
  VINP_FWiperAS_flg : Outport  Port=3
  VINP_FWiperProtection_flg : Outport  Port=4
  wires:
  BHAL_outputs/1 -> [BHAL_outputs]
  inp_CanValid_bus/1 -> [inp_CanValid_bus]
  [BHAL_outputs] -> slr_VHAL_FLTurnLampC_mA/1
  slr_VHAL_FLTurnLampC_mA/1 -> FLTurnLampC/1  "<VHAL_FLTurnLampC_mA>"
  True_VHAL_FLTurnLampC_mA/1 -> FLTurnLampC/2
  [inp_CanValid_bus] -> slr1_1/1
  slr1_1/1 -> FLTurnLampC/3  "<VINP_CANMsgValidGWZoneFR1_flg>"
  FLTurnLampC/1 -> VINP_FLTurnLampC_mA/1  "VINP_FLTurnLampC_mA"
  FLTurnLampC/2 -> Terminator_1/1
  [BHAL_outputs] -> slr_VHAL_FRTurnLampC_mA/1
  slr_VHAL_FRTurnLampC_mA/1 -> FRTurnLampC/1  "<VHAL_FRTurnLampC_mA>"
  True_VHAL_FRTurnLampC_mA/1 -> FRTurnLampC/2
  [inp_CanValid_bus] -> slr1_2/1
  slr1_2/1 -> FRTurnLampC/3  "<VINP_CANMsgValidGWZoneFR1_flg>"
  FRTurnLampC/1 -> VINP_FRTurnLampC_mA/1  "VINP_FRTurnLampC_mA"
  FRTurnLampC/2 -> Terminator_2/1
  [BHAL_outputs] -> slr_VHAL_FWiperAS_flg/1
  slr_VHAL_FWiperAS_flg/1 -> FWiperAS/1  "<VHAL_FWiperAS_flg>"
  True_VHAL_FWiperAS_flg/1 -> FWiperAS/2
  [inp_CanValid_bus] -> slr1_3/1
  slr1_3/1 -> FWiperAS/3  "<VINP_CANMsgValidGWZoneFR1_flg>"
  FWiperAS/1 -> VINP_FWiperAS_flg/1  "VINP_FWiperAS_flg"
  FWiperAS/2 -> Terminator_3/1
  [BHAL_outputs] -> slr_VHAL_FWiperProtection_flg/1
  slr_VHAL_FWiperProtection_flg/1 -> FWiperProtection/1  "<VHAL_FWiperProtection_flg>"
  True_VHAL_FWiperProtection_flg/1 -> FWiperProtection/2
  [inp_CanValid_bus] -> slr1_4/1
  slr1_4/1 -> FWiperProtection/3  "<VINP_CANMsgValidGWZoneFR1_flg>"
  FWiperProtection/1 -> VINP_FWiperProtection_flg/1  "VINP_FWiperProtection_flg"
  FWiperProtection/2 -> Terminator_4/1
